simulink model "waterTankBurner"  (R2014b)
settings: Solver=ode1  StartTime=0.0  StopTime=100  FixedStep=0.0001  MaxStep=0.0001  RelTol=1e-3
(part 3 of 4)

== matlab function waterTankBurner/waterTank4/MATLAB Function ==
  data: q input; ON input; OFF input; x input; qNext output; reset output


function [qNext,reset]  = phi(q,  ON, OFF,x)
%#codegen


if q==1 % q=1, tank is in t1
    if ON==0
        qNext=1;
        reset=0;
    elseif ON==1
        qNext=2;
        reset=1;
    else
        qNext=-1;
        reset=-1;
    end;
    
elseif q==2 % q=2, tank is in t2
    if x<100 && OFF==0
        qNext=2;
        reset=0;
    elseif x>=100
        qNext=3;
        reset=1;
    elseif x<100 && OFF==1
        qNext=4;
        reset=1;
    else
        qNext=-1;
        reset=-1;
    end;

elseif q==3 % q=3, tank is in state t3
    if OFF==0
        qNext=3;
        reset=0;
    elseif OFF==1
        qNext=4;
        reset=1;
    else
        qNext=-1;
        reset=-1;
    end;
elseif q==4 % q=4, tank is in state t4
    if x>20 && ON==0
        qNext=4;
        reset=0;
    elseif x<=20
        qNext=1;
        reset=1;
    elseif x>20 && ON==1
        qNext=2;
        reset=1;
    else
        qNext=-1;
        reset=-1;
    end;
else
    qNext=-1; %this should never execute
    reset=-1;%this should never execute
end

== matlab function waterTankBurner/waterTank4/MATLAB Function1 ==
  data: x input; ode1 output; ode2 output; ode3 output; ode4 output
function [ode1,ode2,ode3,ode4] = ODEs(x)
%#codegen
K=0.075;
h=150;
ode1=0;
ode2=K*(h-x);
ode3=0;
ode4=-K*x;

== matlab function waterTankBurner/waterTank5/MATLAB Function ==
  data: q input; ON input; OFF input; x input; qNext output; reset output


function [qNext,reset]  = phi(q,  ON, OFF,x)
%#codegen


if q==1 % q=1, tank is in t1
    if ON==0
        qNext=1;
        reset=0;
    elseif ON==1
        qNext=2;
        reset=1;
    else
        qNext=-1;
        reset=-1;
    end;
    
elseif q==2 % q=2, tank is in t2
    if x<100 && OFF==0
        qNext=2;
        reset=0;
    elseif x>=100
        qNext=3;
        reset=1;
    elseif x<100 && OFF==1
        qNext=4;
        reset=1;
    else
        qNext=-1;
        reset=-1;
    end;

elseif q==3 % q=3, tank is in state t3
    if OFF==0
        qNext=3;
        reset=0;
    elseif OFF==1
        qNext=4;
        reset=1;
    else
        qNext=-1;
        reset=-1;
    end;
elseif q==4 % q=4, tank is in state t4
    if x>20 && ON==0
        qNext=4;
        reset=0;
    elseif x<=20
        qNext=1;
        reset=1;
    elseif x>20 && ON==1
        qNext=2;
        reset=1;
    else
        qNext=-1;
        reset=-1;
    end;
else
    qNext=-1; %this should never execute
    reset=-1;%this should never execute
end

== matlab function waterTankBurner/waterTank5/MATLAB Function1 ==
  data: x input; ode1 output; ode2 output; ode3 output; ode4 output
function [ode1,ode2,ode3,ode4] = ODEs(x)
%#codegen
K=0.075;
h=150;
ode1=0;
ode2=K*(h-x);
ode3=0;
ode4=-K*x;

== matlab function waterTankBurner/waterTank6/MATLAB Function ==
  data: q input; ON input; OFF input; x input; qNext output; reset output


function [qNext,reset]  = phi(q,  ON, OFF,x)
%#codegen


if q==1 % q=1, tank is in t1
    if ON==0
        qNext=1;
        reset=0;
    elseif ON==1
        qNext=2;
        reset=1;
    else
        qNext=-1;
        reset=-1;
    end;
    
elseif q==2 % q=2, tank is in t2
    if x<100 && OFF==0
        qNext=2;
        reset=0;
    elseif x>=100
        qNext=3;
        reset=1;
    elseif x<100 && OFF==1
        qNext=4;
        reset=1;
    else
        qNext=-1;
        reset=-1;
    end;

elseif q==3 % q=3, tank is in state t3
    if OFF==0
        qNext=3;
        reset=0;
    elseif OFF==1
        qNext=4;
        reset=1;
    else
        qNext=-1;
        reset=-1;
    end;
elseif q==4 % q=4, tank is in state t4
    if x>20 && ON==0
        qNext=4;
        reset=0;
    elseif x<=20
        qNext=1;
        reset=1;
    elseif x>20 && ON==1
        qNext=2;
        reset=1;
    else
        qNext=-1;
        reset=-1;
    end;
else
    qNext=-1; %this should never execute
    reset=-1;%this should never execute
end

== matlab function waterTankBurner/waterTank6/MATLAB Function1 ==
  data: x input; ode1 output; ode2 output; ode3 output; ode4 output
function [ode1,ode2,ode3,ode4] = ODEs(x)
%#codegen
K=0.075;
h=150;
ode1=0;
ode2=K*(h-x);
ode3=0;
ode4=-K*x;

== matlab function waterTankBurner/waterTank7/MATLAB Function ==
  data: q input; ON input; OFF input; x input; qNext output; reset output


function [qNext,reset]  = phi(q,  ON, OFF,x)
%#codegen


if q==1 % q=1, tank is in t1
    if ON==0
        qNext=1;
        reset=0;
    elseif ON==1
        qNext=2;
        reset=1;
    else
        qNext=-1;
        reset=-1;
    end;
    
elseif q==2 % q=2, tank is in t2
    if x<100 && OFF==0
        qNext=2;
        reset=0;
    elseif x>=100
        qNext=3;
        reset=1;
    elseif x<100 && OFF==1
        qNext=4;
        reset=1;
    else
        qNext=-1;
        reset=-1;
    end;

elseif q==3 % q=3, tank is in state t3
    if OFF==0
        qNext=3;
        reset=0;
    elseif OFF==1
        qNext=4;
        reset=1;
    else
        qNext=-1;
        reset=-1;
    end;
elseif q==4 % q=4, tank is in state t4
    if x>20 && ON==0
        qNext=4;
        reset=0;
    elseif x<=20
        qNext=1;
        reset=1;
    elseif x>20 && ON==1
        qNext=2;
        reset=1;
    else
        qNext=-1;
        reset=-1;
    end;
else
    qNext=-1; %this should never execute
    reset=-1;%this should never execute
end

== matlab function waterTankBurner/waterTank7/MATLAB Function1 ==
  data: x input; ode1 output; ode2 output; ode3 output; ode4 output
function [ode1,ode2,ode3,ode4] = ODEs(x)
%#codegen
K=0.075;
h=150;
ode1=0;
ode2=K*(h-x);
ode3=0;
ode4=-K*x;

== matlab function waterTankBurner/waterTank10/MATLAB Function ==
  data: q input; ON input; OFF input; x input; qNext output; reset output


function [qNext,reset]  = phi(q,  ON, OFF,x)
%#codegen


if q==1 % q=1, tank is in t1
    if ON==0
        qNext=1;
        reset=0;
    elseif ON==1
        qNext=2;
        reset=1;
    else
        qNext=-1;
        reset=-1;
    end;
    
elseif q==2 % q=2, tank is in t2
    if x<100 && OFF==0
        qNext=2;
        reset=0;
    elseif x>=100
        qNext=3;
        reset=1;
    elseif x<100 && OFF==1
        qNext=4;
        reset=1;
    else
        qNext=-1;
        reset=-1;
    end;

elseif q==3 % q=3, tank is in state t3
    if OFF==0
        qNext=3;
        reset=0;
    elseif OFF==1
        qNext=4;
        reset=1;
    else
        qNext=-1;
        reset=-1;
    end;
elseif q==4 % q=4, tank is in state t4
    if x>20 && ON==0
        qNext=4;
        reset=0;
    elseif x<=20
        qNext=1;
        reset=1;
    elseif x>20 && ON==1
        qNext=2;
        reset=1;
    else
        qNext=-1;
        reset=-1;
    end;
else
    qNext=-1; %this should never execute
    reset=-1;%this should never execute
end

== matlab function waterTankBurner/waterTank10/MATLAB Function1 ==
  data: x input; ode1 output; ode2 output; ode3 output; ode4 output
function [ode1,ode2,ode3,ode4] = ODEs(x)
%#codegen
K=0.075;
h=150;
ode1=0;
ode2=K*(h-x);
ode3=0;
ode4=-K*x;

== matlab function waterTankBurner/waterTank11/MATLAB Function ==
  data: q input; ON input; OFF input; x input; qNext output; reset output


function [qNext,reset]  = phi(q,  ON, OFF,x)
%#codegen


if q==1 % q=1, tank is in t1
    if ON==0
        qNext=1;
        reset=0;
    elseif ON==1
        qNext=2;
        reset=1;
    else
        qNext=-1;
        reset=-1;
    end;
    
elseif q==2 % q=2, tank is in t2
    if x<100 && OFF==0
        qNext=2;
        reset=0;
    elseif x>=100
        qNext=3;
        reset=1;
    elseif x<100 && OFF==1
        qNext=4;
        reset=1;
    else
        qNext=-1;
        reset=-1;
    end;

elseif q==3 % q=3, tank is in state t3
    if OFF==0
        qNext=3;
        reset=0;
    elseif OFF==1
        qNext=4;
        reset=1;
    else
        qNext=-1;
        reset=-1;
    end;
elseif q==4 % q=4, tank is in state t4
    if x>20 && ON==0
        qNext=4;
        reset=0;
    elseif x<=20
        qNext=1;
        reset=1;
    elseif x>20 && ON==1
        qNext=2;
        reset=1;
    else
        qNext=-1;
        reset=-1;
    end;
else
    qNext=-1; %this should never execute
    reset=-1;%this should never execute
end

== matlab function waterTankBurner/waterTank11/MATLAB Function1 ==
  data: x input; ode1 output; ode2 output; ode3 output; ode4 output
function [ode1,ode2,ode3,ode4] = ODEs(x)
%#codegen
K=0.075;
h=150;
ode1=0;
ode2=K*(h-x);
ode3=0;
ode4=-K*x;

== matlab function waterTankBurner/waterTank8/MATLAB Function ==
  data: q input; ON input; OFF input; x input; qNext output; reset output


function [qNext,reset]  = phi(q,  ON, OFF,x)
%#codegen


if q==1 % q=1, tank is in t1
    if ON==0
        qNext=1;
        reset=0;
    elseif ON==1
        qNext=2;
        reset=1;
    else
        qNext=-1;
        reset=-1;
    end;
    
elseif q==2 % q=2, tank is in t2
    if x<100 && OFF==0
        qNext=2;
        reset=0;
    elseif x>=100
        qNext=3;
        reset=1;
    elseif x<100 && OFF==1
        qNext=4;
        reset=1;
    else
        qNext=-1;
        reset=-1;
    end;

elseif q==3 % q=3, tank is in state t3
    if OFF==0
        qNext=3;
        reset=0;
    elseif OFF==1
        qNext=4;
        reset=1;
    else
        qNext=-1;
        reset=-1;
    end;
elseif q==4 % q=4, tank is in state t4
    if x>20 && ON==0
        qNext=4;
        reset=0;
    elseif x<=20
        qNext=1;
        reset=1;
    elseif x>20 && ON==1
        qNext=2;
        reset=1;
    else
        qNext=-1;
        reset=-1;
    end;
else
    qNext=-1; %this should never execute
    reset=-1;%this should never execute
end

== matlab function waterTankBurner/waterTank8/MATLAB Function1 ==
  data: x input; ode1 output; ode2 output; ode3 output; ode4 output
function [ode1,ode2,ode3,ode4] = ODEs(x)
%#codegen
K=0.075;
h=150;
ode1=0;
ode2=K*(h-x);
ode3=0;
ode4=-K*x;

== matlab function waterTankBurner/waterTank9/MATLAB Function ==
  data: q input; ON input; OFF input; x input; qNext output; reset output


function [qNext,reset]  = phi(q,  ON, OFF,x)
%#codegen


if q==1 % q=1, tank is in t1
    if ON==0
        qNext=1;
        reset=0;
    elseif ON==1
        qNext=2;
        reset=1;
    else
        qNext=-1;
        reset=-1;
    end;
    
elseif q==2 % q=2, tank is in t2
    if x<100 && OFF==0
        qNext=2;
        reset=0;
    elseif x>=100
        qNext=3;
        reset=1;
    elseif x<100 && OFF==1
        qNext=4;
        reset=1;
    else
        qNext=-1;
        reset=-1;
    end;

elseif q==3 % q=3, tank is in state t3
    if OFF==0
        qNext=3;
        reset=0;
    elseif OFF==1
        qNext=4;
        reset=1;
    else
        qNext=-1;
        reset=-1;
    end;
elseif q==4 % q=4, tank is in state t4
    if x>20 && ON==0
        qNext=4;
        reset=0;
    elseif x<=20
        qNext=1;
        reset=1;
    elseif x>20 && ON==1
        qNext=2;
        reset=1;
    else
        qNext=-1;
        reset=-1;
    end;
else
    qNext=-1; %this should never execute
    reset=-1;%this should never execute
end

== matlab function waterTankBurner/waterTank9/MATLAB Function1 ==
  data: x input; ode1 output; ode2 output; ode3 output; ode4 output
function [ode1,ode2,ode3,ode4] = ODEs(x)
%#codegen
K=0.075;
h=150;
ode1=0;
ode2=K*(h-x);
ode3=0;
ode4=-K*x;

== matlab function waterTankBurner/waterTank12/MATLAB Function ==
  data: q input; ON input; OFF input; x input; qNext output; reset output


function [qNext,reset]  = phi(q,  ON, OFF,x)
%#codegen


if q==1 % q=1, tank is in t1
    if ON==0
        qNext=1;
        reset=0;
    elseif ON==1
        qNext=2;
        reset=1;
    else
        qNext=-1;
        reset=-1;
    end;
    
elseif q==2 % q=2, tank is in t2
    if x<100 && OFF==0
        qNext=2;
        reset=0;
    elseif x>=100
        qNext=3;
        reset=1;
    elseif x<100 && OFF==1
        qNext=4;
        reset=1;
    else
        qNext=-1;
        reset=-1;
    end;

elseif q==3 % q=3, tank is in state t3
    if OFF==0
        qNext=3;
        reset=0;
    elseif OFF==1
        qNext=4;
        reset=1;
    else
        qNext=-1;
        reset=-1;
    end;
elseif q==4 % q=4, tank is in state t4
    if x>20 && ON==0
        qNext=4;
        reset=0;
    elseif x<=20
        qNext=1;
        reset=1;
    elseif x>20 && ON==1
        qNext=2;
        reset=1;
    else
        qNext=-1;
        reset=-1;
    end;
else
    qNext=-1; %this should never execute
    reset=-1;%this should never execute
end

== matlab function waterTankBurner/waterTank12/MATLAB Function1 ==
  data: x input; ode1 output; ode2 output; ode3 output; ode4 output
function [ode1,ode2,ode3,ode4] = ODEs(x)
%#codegen
K=0.075;
h=150;
ode1=0;
ode2=K*(h-x);
ode3=0;
ode4=-K*x;

== matlab function waterTankBurner/waterTank13/MATLAB Function ==
  data: q input; ON input; OFF input; x input; qNext output; reset output


function [qNext,reset]  = phi(q,  ON, OFF,x)
%#codegen


if q==1 % q=1, tank is in t1
    if ON==0
        qNext=1;
        reset=0;
    elseif ON==1
        qNext=2;
        reset=1;
    else
        qNext=-1;
        reset=-1;
    end;
    
elseif q==2 % q=2, tank is in t2
    if x<100 && OFF==0
        qNext=2;
        reset=0;
    elseif x>=100
        qNext=3;
        reset=1;
    elseif x<100 && OFF==1
        qNext=4;
        reset=1;
    else
        qNext=-1;
        reset=-1;
    end;

elseif q==3 % q=3, tank is in state t3
    if OFF==0
        qNext=3;
        reset=0;
    elseif OFF==1
        qNext=4;
        reset=1;
    else
        qNext=-1;
        reset=-1;
    end;
elseif q==4 % q=4, tank is in state t4
    if x>20 && ON==0
        qNext=4;
        reset=0;
    elseif x<=20
        qNext=1;
        reset=1;
    elseif x>20 && ON==1
        qNext=2;
        reset=1;
    else
        qNext=-1;
        reset=-1;
    end;
else
    qNext=-1; %this should never execute
    reset=-1;%this should never execute
end

== matlab function waterTankBurner/waterTank13/MATLAB Function1 ==
  data: x input; ode1 output; ode2 output; ode3 output; ode4 output
function [ode1,ode2,ode3,ode4] = ODEs(x)
%#codegen
K=0.075;
h=150;
ode1=0;
ode2=K*(h-x);
ode3=0;
ode4=-K*x;

== matlab function waterTankBurner/waterTank14/MATLAB Function ==
  data: q input; ON input; OFF input; x input; qNext output; reset output


function [qNext,reset]  = phi(q,  ON, OFF,x)
%#codegen


if q==1 % q=1, tank is in t1
    if ON==0
        qNext=1;
        reset=0;
    elseif ON==1
        qNext=2;
        reset=1;
    else
        qNext=-1;
        reset=-1;
    end;
    
elseif q==2 % q=2, tank is in t2
    if x<100 && OFF==0
        qNext=2;
        reset=0;
    elseif x>=100
        qNext=3;
        reset=1;
    elseif x<100 && OFF==1
        qNext=4;
        reset=1;
    else
        qNext=-1;
        reset=-1;
    end;

elseif q==3 % q=3, tank is in state t3
    if OFF==0
        qNext=3;
        reset=0;
    elseif OFF==1
        qNext=4;
        reset=1;
    else
        qNext=-1;
        reset=-1;
    end;
elseif q==4 % q=4, tank is in state t4
    if x>20 && ON==0
        qNext=4;
        reset=0;
    elseif x<=20
        qNext=1;
        reset=1;
    elseif x>20 && ON==1
        qNext=2;
        reset=1;
    else
        qNext=-1;
        reset=-1;
    end;
else
    qNext=-1; %this should never execute
    reset=-1;%this should never execute
end

== matlab function waterTankBurner/waterTank14/MATLAB Function1 ==
  data: x input; ode1 output; ode2 output; ode3 output; ode4 output
function [ode1,ode2,ode3,ode4] = ODEs(x)
%#codegen
K=0.075;
h=150;
ode1=0;
ode2=K*(h-x);
ode3=0;
ode4=-K*x;

== matlab function waterTankBurner/waterTank15/MATLAB Function ==
  data: q input; ON input; OFF input; x input; qNext output; reset output


function [qNext,reset]  = phi(q,  ON, OFF,x)
%#codegen


if q==1 % q=1, tank is in t1
    if ON==0
        qNext=1;
        reset=0;
    elseif ON==1
        qNext=2;
        reset=1;
    else
        qNext=-1;
        reset=-1;
    end;
    
elseif q==2 % q=2, tank is in t2
    if x<100 && OFF==0
        qNext=2;
        reset=0;
    elseif x>=100
        qNext=3;
        reset=1;
    elseif x<100 && OFF==1
        qNext=4;
        reset=1;
    else
        qNext=-1;
        reset=-1;
    end;

elseif q==3 % q=3, tank is in state t3
    if OFF==0
        qNext=3;
        reset=0;
    elseif OFF==1
        qNext=4;
        reset=1;
    else
        qNext=-1;
        reset=-1;
    end;
elseif q==4 % q=4, tank is in state t4
    if x>20 && ON==0
        qNext=4;
        reset=0;
    elseif x<=20
        qNext=1;
        reset=1;
    elseif x>20 && ON==1
        qNext=2;
        reset=1;
    else
        qNext=-1;
        reset=-1;
    end;
else
    qNext=-1; %this should never execute
    reset=-1;%this should never execute
end

== matlab function waterTankBurner/waterTank15/MATLAB Function1 ==
  data: x input; ode1 output; ode2 output; ode3 output; ode4 output
function [ode1,ode2,ode3,ode4] = ODEs(x)
%#codegen
K=0.075;
h=150;
ode1=0;
ode2=K*(h-x);
ode3=0;
ode4=-K*x;

== matlab function waterTankBurner/waterTank16/MATLAB Function ==
  data: q input; ON input; OFF input; x input; qNext output; reset output


function [qNext,reset]  = phi(q,  ON, OFF,x)
%#codegen


if q==1 % q=1, tank is in t1
    if ON==0
        qNext=1;
        reset=0;
    elseif ON==1
        qNext=2;
        reset=1;
    else
        qNext=-1;
        reset=-1;
    end;
    
elseif q==2 % q=2, tank is in t2
    if x<100 && OFF==0
        qNext=2;
        reset=0;
    elseif x>=100
        qNext=3;
        reset=1;
    elseif x<100 && OFF==1
        qNext=4;
        reset=1;
    else
        qNext=-1;
        reset=-1;
    end;

elseif q==3 % q=3, tank is in state t3
    if OFF==0
        qNext=3;
        reset=0;
    elseif OFF==1
        qNext=4;
        reset=1;
    else
        qNext=-1;
        reset=-1;
    end;
elseif q==4 % q=4, tank is in state t4
    if x>20 && ON==0
        qNext=4;
        reset=0;
    elseif x<=20
        qNext=1;
        reset=1;
    elseif x>20 && ON==1
        qNext=2;
        reset=1;
    else
        qNext=-1;
        reset=-1;
    end;
else
    qNext=-1; %this should never execute
    reset=-1;%this should never execute
end

== matlab function waterTankBurner/waterTank16/MATLAB Function1 ==
  data: x input; ode1 output; ode2 output; ode3 output; ode4 output
function [ode1,ode2,ode3,ode4] = ODEs(x)
%#codegen
K=0.075;
h=150;
ode1=0;
ode2=K*(h-x);
ode3=0;
ode4=-K*x;

== matlab function waterTankBurner/waterTank17/MATLAB Function ==
  data: q input; ON input; OFF input; x input; qNext output; reset output


function [qNext,reset]  = phi(q,  ON, OFF,x)
%#codegen


if q==1 % q=1, tank is in t1
    if ON==0
        qNext=1;
        reset=0;
    elseif ON==1
        qNext=2;
        reset=1;
    else
        qNext=-1;
        reset=-1;
    end;
    
elseif q==2 % q=2, tank is in t2
    if x<100 && OFF==0
        qNext=2;
        reset=0;
    elseif x>=100
        qNext=3;
        reset=1;
    elseif x<100 && OFF==1
        qNext=4;
        reset=1;
    else
        qNext=-1;
        reset=-1;
    end;

elseif q==3 % q=3, tank is in state t3
    if OFF==0
        qNext=3;
        reset=0;
    elseif OFF==1
        qNext=4;
        reset=1;
    else
        qNext=-1;
        reset=-1;
    end;
elseif q==4 % q=4, tank is in state t4
    if x>20 && ON==0
        qNext=4;
        reset=0;
    elseif x<=20
        qNext=1;
        reset=1;
    elseif x>20 && ON==1
        qNext=2;
        reset=1;
    else
        qNext=-1;
        reset=-1;
    end;
else
    qNext=-1; %this should never execute
    reset=-1;%this should never execute
end

== matlab function waterTankBurner/waterTank17/MATLAB Function1 ==
  data: x input; ode1 output; ode2 output; ode3 output; ode4 output
function [ode1,ode2,ode3,ode4] = ODEs(x)
%#codegen
K=0.075;
h=150;
ode1=0;
ode2=K*(h-x);
ode3=0;
ode4=-K*x;

== matlab function waterTankBurner/waterTank18/MATLAB Function ==
  data: q input; ON input; OFF input; x input; qNext output; reset output


function [qNext,reset]  = phi(q,  ON, OFF,x)
%#codegen


if q==1 % q=1, tank is in t1
    if ON==0
        qNext=1;
        reset=0;
    elseif ON==1
        qNext=2;
        reset=1;
    else
        qNext=-1;
        reset=-1;
    end;
    
elseif q==2 % q=2, tank is in t2
    if x<100 && OFF==0
        qNext=2;
        reset=0;
    elseif x>=100
        qNext=3;
        reset=1;
    elseif x<100 && OFF==1
        qNext=4;
        reset=1;
    else
        qNext=-1;
        reset=-1;
    end;

elseif q==3 % q=3, tank is in state t3
    if OFF==0
        qNext=3;
        reset=0;
    elseif OFF==1
        qNext=4;
        reset=1;
    else
        qNext=-1;
        reset=-1;
    end;
elseif q==4 % q=4, tank is in state t4
    if x>20 && ON==0
        qNext=4;
        reset=0;
    elseif x<=20
        qNext=1;
        reset=1;
    elseif x>20 && ON==1
        qNext=2;
        reset=1;
    else
        qNext=-1;
        reset=-1;
    end;
else
    qNext=-1; %this should never execute
    reset=-1;%this should never execute
end

== matlab function waterTankBurner/waterTank18/MATLAB Function1 ==
  data: x input; ode1 output; ode2 output; ode3 output; ode4 output
function [ode1,ode2,ode3,ode4] = ODEs(x)
%#codegen
K=0.075;
h=150;
ode1=0;
ode2=K*(h-x);
ode3=0;
ode4=-K*x;

== matlab function waterTankBurner/waterTank19/MATLAB Function ==
  data: q input; ON input; OFF input; x input; qNext output; reset output


function [qNext,reset]  = phi(q,  ON, OFF,x)
%#codegen


if q==1 % q=1, tank is in t1
    if ON==0
        qNext=1;
        reset=0;
    elseif ON==1
        qNext=2;
        reset=1;
    else
        qNext=-1;
        reset=-1;
    end;
    
elseif q==2 % q=2, tank is in t2
    if x<100 && OFF==0
        qNext=2;
        reset=0;
    elseif x>=100
        qNext=3;
        reset=1;
    elseif x<100 && OFF==1
        qNext=4;
        reset=1;
    else
        qNext=-1;
        reset=-1;
    end;

elseif q==3 % q=3, tank is in state t3
    if OFF==0
        qNext=3;
        reset=0;
    elseif OFF==1
        qNext=4;
        reset=1;
    else
        qNext=-1;
        reset=-1;
    end;
elseif q==4 % q=4, tank is in state t4
    if x>20 && ON==0
        qNext=4;
        reset=0;
    elseif x<=20
        qNext=1;
        reset=1;
    elseif x>20 && ON==1
        qNext=2;
        reset=1;
    else
        qNext=-1;
        reset=-1;
    end;
else
    qNext=-1; %this should never execute
    reset=-1;%this should never execute
end

== matlab function waterTankBurner/waterTank19/MATLAB Function1 ==
  data: x input; ode1 output; ode2 output; ode3 output; ode4 output
function [ode1,ode2,ode3,ode4] = ODEs(x)
%#codegen
K=0.075;
h=150;
ode1=0;
ode2=K*(h-x);
ode3=0;
ode4=-K*x;

== matlab function waterTankBurner/waterTank20/MATLAB Function ==
  data: q input; ON input; OFF input; x input; qNext output; reset output


function [qNext,reset]  = phi(q,  ON, OFF,x)
%#codegen


if q==1 % q=1, tank is in t1
    if ON==0
        qNext=1;
        reset=0;
    elseif ON==1
        qNext=2;
        reset=1;
    else
        qNext=-1;
        reset=-1;
    end;
    
elseif q==2 % q=2, tank is in t2
    if x<100 && OFF==0
        qNext=2;
        reset=0;
    elseif x>=100
        qNext=3;
        reset=1;
    elseif x<100 && OFF==1
        qNext=4;
        reset=1;
    else
        qNext=-1;
        reset=-1;
    end;

elseif q==3 % q=3, tank is in state t3
    if OFF==0
        qNext=3;
        reset=0;
    elseif OFF==1
        qNext=4;
        reset=1;
    else
        qNext=-1;
        reset=-1;
    end;
elseif q==4 % q=4, tank is in state t4
    if x>20 && ON==0
        qNext=4;
        reset=0;
    elseif x<=20
        qNext=1;
        reset=1;
    elseif x>20 && ON==1
        qNext=2;
        reset=1;
    else
        qNext=-1;
        reset=-1;
    end;
else
    qNext=-1; %this should never execute
    reset=-1;%this should never execute
end

== matlab function waterTankBurner/waterTank20/MATLAB Function1 ==
  data: x input; ode1 output; ode2 output; ode3 output; ode4 output
function [ode1,ode2,ode3,ode4] = ODEs(x)
%#codegen
K=0.075;
h=150;
ode1=0;
ode2=K*(h-x);
ode3=0;
ode4=-K*x;

== matlab function waterTankBurner/waterTank21/MATLAB Function ==
  data: q input; ON input; OFF input; x input; qNext output; reset output


function [qNext,reset]  = phi(q,  ON, OFF,x)
%#codegen


if q==1 % q=1, tank is in t1
    if ON==0
        qNext=1;
        reset=0;
    elseif ON==1
        qNext=2;
        reset=1;
    else
        qNext=-1;
        reset=-1;
    end;
    
elseif q==2 % q=2, tank is in t2
    if x<100 && OFF==0
        qNext=2;
        reset=0;
    elseif x>=100
        qNext=3;
        reset=1;
    elseif x<100 && OFF==1
        qNext=4;
        reset=1;
    else
        qNext=-1;
        reset=-1;
    end;

elseif q==3 % q=3, tank is in state t3
    if OFF==0
        qNext=3;
        reset=0;
    elseif OFF==1
        qNext=4;
        reset=1;
    else
        qNext=-1;
        reset=-1;
    end;
elseif q==4 % q=4, tank is in state t4
    if x>20 && ON==0
        qNext=4;
        reset=0;
    elseif x<=20
        qNext=1;
        reset=1;
    elseif x>20 && ON==1
        qNext=2;
        reset=1;
    else
        qNext=-1;
        reset=-1;
    end;
else
    qNext=-1; %this should never execute
    reset=-1;%this should never execute
end

== matlab function waterTankBurner/waterTank21/MATLAB Function1 ==
  data: x input; ode1 output; ode2 output; ode3 output; ode4 output
function [ode1,ode2,ode3,ode4] = ODEs(x)
%#codegen
K=0.075;
h=150;
ode1=0;
ode2=K*(h-x);
ode3=0;
ode4=-K*x;

== matlab function waterTankBurner/waterTank22/MATLAB Function ==
  data: q input; ON input; OFF input; x input; qNext output; reset output


function [qNext,reset]  = phi(q,  ON, OFF,x)
%#codegen


if q==1 % q=1, tank is in t1
    if ON==0
        qNext=1;
        reset=0;
    elseif ON==1
        qNext=2;
        reset=1;
    else
        qNext=-1;
        reset=-1;
    end;
    
elseif q==2 % q=2, tank is in t2
    if x<100 && OFF==0
        qNext=2;
        reset=0;
    elseif x>=100
        qNext=3;
        reset=1;
    elseif x<100 && OFF==1
        qNext=4;
        reset=1;
    else
        qNext=-1;
        reset=-1;
    end;

elseif q==3 % q=3, tank is in state t3
    if OFF==0
        qNext=3;
        reset=0;
    elseif OFF==1
        qNext=4;
        reset=1;
    else
        qNext=-1;
        reset=-1;
    end;
elseif q==4 % q=4, tank is in state t4
    if x>20 && ON==0
        qNext=4;
        reset=0;
    elseif x<=20
        qNext=1;
        reset=1;
    elseif x>20 && ON==1
        qNext=2;
        reset=1;
    else
        qNext=-1;
        reset=-1;
    end;
else
    qNext=-1; %this should never execute
    reset=-1;%this should never execute
end

== matlab function waterTankBurner/waterTank22/MATLAB Function1 ==
  data: x input; ode1 output; ode2 output; ode3 output; ode4 output
function [ode1,ode2,ode3,ode4] = ODEs(x)
%#codegen
K=0.075;
h=150;
ode1=0;
ode2=K*(h-x);
ode3=0;
ode4=-K*x;

== matlab function waterTankBurner/waterTank23/MATLAB Function ==
  data: q input; ON input; OFF input; x input; qNext output; reset output


function [qNext,reset]  = phi(q,  ON, OFF,x)
%#codegen


if q==1 % q=1, tank is in t1
    if ON==0
        qNext=1;
        reset=0;
    elseif ON==1
        qNext=2;
        reset=1;
    else
        qNext=-1;
        reset=-1;
    end;
    
elseif q==2 % q=2, tank is in t2
    if x<100 && OFF==0
        qNext=2;
        reset=0;
    elseif x>=100
        qNext=3;
        reset=1;
    elseif x<100 && OFF==1
        qNext=4;
        reset=1;
    else
        qNext=-1;
        reset=-1;
    end;

elseif q==3 % q=3, tank is in state t3
    if OFF==0
        qNext=3;
        reset=0;
    elseif OFF==1
        qNext=4;
        reset=1;
    else
        qNext=-1;
        reset=-1;
    end;
elseif q==4 % q=4, tank is in state t4
    if x>20 && ON==0
        qNext=4;
        reset=0;
    elseif x<=20
        qNext=1;
        reset=1;
    elseif x>20 && ON==1
        qNext=2;
        reset=1;
    else
        qNext=-1;
        reset=-1;
    end;
else
    qNext=-1; %this should never execute
    reset=-1;%this should never execute
end

== matlab function waterTankBurner/waterTank23/MATLAB Function1 ==
  data: x input; ode1 output; ode2 output; ode3 output; ode4 output
function [ode1,ode2,ode3,ode4] = ODEs(x)
%#codegen
K=0.075;
h=150;
ode1=0;
ode2=K*(h-x);
ode3=0;
ode4=-K*x;

== matlab function waterTankBurner/waterTank24/MATLAB Function ==
  data: q input; ON input; OFF input; x input; qNext output; reset output


function [qNext,reset]  = phi(q,  ON, OFF,x)
%#codegen


if q==1 % q=1, tank is in t1
    if ON==0
        qNext=1;
        reset=0;
    elseif ON==1
        qNext=2;
        reset=1;
    else
        qNext=-1;
        reset=-1;
    end;
    
elseif q==2 % q=2, tank is in t2
    if x<100 && OFF==0
        qNext=2;
        reset=0;
    elseif x>=100
        qNext=3;
        reset=1;
    elseif x<100 && OFF==1
        qNext=4;
        reset=1;
    else
        qNext=-1;
        reset=-1;
    end;

elseif q==3 % q=3, tank is in state t3
    if OFF==0
        qNext=3;
        reset=0;
    elseif OFF==1
        qNext=4;
        reset=1;
    else
        qNext=-1;
        reset=-1;
    end;
elseif q==4 % q=4, tank is in state t4
    if x>20 && ON==0
        qNext=4;
        reset=0;
    elseif x<=20
        qNext=1;
        reset=1;
    elseif x>20 && ON==1
        qNext=2;
        reset=1;
    else
        qNext=-1;
        reset=-1;
    end;
else
    qNext=-1; %this should never execute
    reset=-1;%this should never execute
end

== matlab function waterTankBurner/waterTank24/MATLAB Function1 ==
  data: x input; ode1 output; ode2 output; ode3 output; ode4 output
function [ode1,ode2,ode3,ode4] = ODEs(x)
%#codegen
K=0.075;
h=150;
ode1=0;
ode2=K*(h-x);
ode3=0;
ode4=-K*x;

== matlab function waterTankBurner/waterTank25/MATLAB Function ==
  data: q input; ON input; OFF input; x input; qNext output; reset output


function [qNext,reset]  = phi(q,  ON, OFF,x)
%#codegen


if q==1 % q=1, tank is in t1
    if ON==0
        qNext=1;
        reset=0;
    elseif ON==1
        qNext=2;
        reset=1;
    else
        qNext=-1;
        reset=-1;
    end;
    
elseif q==2 % q=2, tank is in t2
    if x<100 && OFF==0
        qNext=2;
        reset=0;
    elseif x>=100
        qNext=3;
        reset=1;
    elseif x<100 && OFF==1
        qNext=4;
        reset=1;
    else
        qNext=-1;
        reset=-1;
    end;

elseif q==3 % q=3, tank is in state t3
    if OFF==0
        qNext=3;
        reset=0;
    elseif OFF==1
        qNext=4;
        reset=1;
    else
        qNext=-1;
        reset=-1;
    end;
elseif q==4 % q=4, tank is in state t4
    if x>20 && ON==0
        qNext=4;
        reset=0;
    elseif x<=20
        qNext=1;
        reset=1;
    elseif x>20 && ON==1
        qNext=2;
        reset=1;
    else
        qNext=-1;
        reset=-1;
    end;
else
    qNext=-1; %this should never execute
    reset=-1;%this should never execute
end

== matlab function waterTankBurner/waterTank25/MATLAB Function1 ==
  data: x input; ode1 output; ode2 output; ode3 output; ode4 output
function [ode1,ode2,ode3,ode4] = ODEs(x)
%#codegen
K=0.075;
h=150;
ode1=0;
ode2=K*(h-x);
ode3=0;
ode4=-K*x;

== matlab function waterTankBurner/waterTank26/MATLAB Function ==
  data: q input; ON input; OFF input; x input; qNext output; reset output


function [qNext,reset]  = phi(q,  ON, OFF,x)
%#codegen


if q==1 % q=1, tank is in t1
    if ON==0
        qNext=1;
        reset=0;
    elseif ON==1
        qNext=2;
        reset=1;
    else
        qNext=-1;
        reset=-1;
    end;
    
elseif q==2 % q=2, tank is in t2
    if x<100 && OFF==0
        qNext=2;
        reset=0;
    elseif x>=100
        qNext=3;
        reset=1;
    elseif x<100 && OFF==1
        qNext=4;
        reset=1;
    else
        qNext=-1;
        reset=-1;
    end;

elseif q==3 % q=3, tank is in state t3
    if OFF==0
        qNext=3;
        reset=0;
    elseif OFF==1
        qNext=4;
        reset=1;
    else
        qNext=-1;
        reset=-1;
    end;
elseif q==4 % q=4, tank is in state t4
    if x>20 && ON==0
        qNext=4;
        reset=0;
    elseif x<=20
        qNext=1;
        reset=1;
    elseif x>20 && ON==1
        qNext=2;
        reset=1;
    else
        qNext=-1;
        reset=-1;
    end;
else
    qNext=-1; %this should never execute
    reset=-1;%this should never execute
end

== matlab function waterTankBurner/waterTank26/MATLAB Function1 ==
  data: x input; ode1 output; ode2 output; ode3 output; ode4 output
function [ode1,ode2,ode3,ode4] = ODEs(x)
%#codegen
K=0.075;
h=150;
ode1=0;
ode2=K*(h-x);
ode3=0;
ode4=-K*x;

== matlab function waterTankBurner/waterTank27/MATLAB Function ==
  data: q input; ON input; OFF input; x input; qNext output; reset output


function [qNext,reset]  = phi(q,  ON, OFF,x)
%#codegen


if q==1 % q=1, tank is in t1
    if ON==0
        qNext=1;
        reset=0;
    elseif ON==1
        qNext=2;
        reset=1;
    else
        qNext=-1;
        reset=-1;
    end;
    
elseif q==2 % q=2, tank is in t2
    if x<100 && OFF==0
        qNext=2;
        reset=0;
    elseif x>=100
        qNext=3;
        reset=1;
    elseif x<100 && OFF==1
        qNext=4;
        reset=1;
    else
        qNext=-1;
        reset=-1;
    end;

elseif q==3 % q=3, tank is in state t3
    if OFF==0
        qNext=3;
        reset=0;
    elseif OFF==1
        qNext=4;
        reset=1;
    else
        qNext=-1;
        reset=-1;
    end;
elseif q==4 % q=4, tank is in state t4
    if x>20 && ON==0
        qNext=4;
        reset=0;
    elseif x<=20
        qNext=1;
        reset=1;
    elseif x>20 && ON==1
        qNext=2;
        reset=1;
    else
        qNext=-1;
        reset=-1;
    end;
else
    qNext=-1; %this should never execute
    reset=-1;%this should never execute
end

== matlab function waterTankBurner/waterTank27/MATLAB Function1 ==
  data: x input; ode1 output; ode2 output; ode3 output; ode4 output
function [ode1,ode2,ode3,ode4] = ODEs(x)
%#codegen
K=0.075;
h=150;
ode1=0;
ode2=K*(h-x);
ode3=0;
ode4=-K*x;

== matlab function waterTankBurner/waterTank28/MATLAB Function ==
  data: q input; ON input; OFF input; x input; qNext output; reset output


function [qNext,reset]  = phi(q,  ON, OFF,x)
%#codegen


if q==1 % q=1, tank is in t1
    if ON==0
        qNext=1;
        reset=0;
    elseif ON==1
        qNext=2;
        reset=1;
    else
        qNext=-1;
        reset=-1;
    end;
    
elseif q==2 % q=2, tank is in t2
    if x<100 && OFF==0
        qNext=2;
        reset=0;
    elseif x>=100
        qNext=3;
        reset=1;
    elseif x<100 && OFF==1
        qNext=4;
        reset=1;
    else
        qNext=-1;
        reset=-1;
    end;

elseif q==3 % q=3, tank is in state t3
    if OFF==0
        qNext=3;
        reset=0;
    elseif OFF==1
        qNext=4;
        reset=1;
    else
        qNext=-1;
        reset=-1;
    end;
elseif q==4 % q=4, tank is in state t4
    if x>20 && ON==0
        qNext=4;
        reset=0;
    elseif x<=20
        qNext=1;
        reset=1;
    elseif x>20 && ON==1
        qNext=2;
        reset=1;
    else
        qNext=-1;
        reset=-1;
    end;
else
    qNext=-1; %this should never execute
    reset=-1;%this should never execute
end

== matlab function waterTankBurner/waterTank28/MATLAB Function1 ==
  data: x input; ode1 output; ode2 output; ode3 output; ode4 output
function [ode1,ode2,ode3,ode4] = ODEs(x)
%#codegen
K=0.075;
h=150;
ode1=0;
ode2=K*(h-x);
ode3=0;
ode4=-K*x;

== matlab function waterTankBurner/waterTank29/MATLAB Function ==
  data: q input; ON input; OFF input; x input; qNext output; reset output


function [qNext,reset]  = phi(q,  ON, OFF,x)
%#codegen


if q==1 % q=1, tank is in t1
    if ON==0
        qNext=1;
        reset=0;
    elseif ON==1
        qNext=2;
        reset=1;
    else
        qNext=-1;
        reset=-1;
    end;
    
elseif q==2 % q=2, tank is in t2
    if x<100 && OFF==0
        qNext=2;
        reset=0;
    elseif x>=100
        qNext=3;
        reset=1;
    elseif x<100 && OFF==1
        qNext=4;
        reset=1;
    else
        qNext=-1;
        reset=-1;
    end;

elseif q==3 % q=3, tank is in state t3
    if OFF==0
        qNext=3;
        reset=0;
    elseif OFF==1
        qNext=4;
        reset=1;
    else
        qNext=-1;
        reset=-1;
    end;
elseif q==4 % q=4, tank is in state t4
    if x>20 && ON==0
        qNext=4;
        reset=0;
    elseif x<=20
        qNext=1;
        reset=1;
    elseif x>20 && ON==1
        qNext=2;
        reset=1;
    else
        qNext=-1;
        reset=-1;
    end;
else
    qNext=-1; %this should never execute
    reset=-1;%this should never execute
end

== matlab function waterTankBurner/waterTank29/MATLAB Function1 ==
  data: x input; ode1 output; ode2 output; ode3 output; ode4 output
function [ode1,ode2,ode3,ode4] = ODEs(x)
%#codegen
K=0.075;
h=150;
ode1=0;
ode2=K*(h-x);
ode3=0;
ode4=-K*x;

== matlab function waterTankBurner/waterTank30/MATLAB Function ==
  data: q input; ON input; OFF input; x input; qNext output; reset output


function [qNext,reset]  = phi(q,  ON, OFF,x)
%#codegen


if q==1 % q=1, tank is in t1
    if ON==0
        qNext=1;
        reset=0;
    elseif ON==1
        qNext=2;
        reset=1;
    else
        qNext=-1;
        reset=-1;
    end;
    
elseif q==2 % q=2, tank is in t2
    if x<100 && OFF==0
        qNext=2;
        reset=0;
    elseif x>=100
        qNext=3;
        reset=1;
    elseif x<100 && OFF==1
        qNext=4;
        reset=1;
    else
        qNext=-1;
        reset=-1;
    end;

elseif q==3 % q=3, tank is in state t3
    if OFF==0
        qNext=3;
        reset=0;
    elseif OFF==1
        qNext=4;
        reset=1;
    else
        qNext=-1;
        reset=-1;
    end;
elseif q==4 % q=4, tank is in state t4
    if x>20 && ON==0
        qNext=4;
        reset=0;
    elseif x<=20
        qNext=1;
        reset=1;
    elseif x>20 && ON==1
        qNext=2;
        reset=1;
    else
        qNext=-1;
        reset=-1;
    end;
else
    qNext=-1; %this should never execute
    reset=-1;%this should never execute
end

== matlab function waterTankBurner/waterTank30/MATLAB Function1 ==
  data: x input; ode1 output; ode2 output; ode3 output; ode4 output
function [ode1,ode2,ode3,ode4] = ODEs(x)
%#codegen
K=0.075;
h=150;
ode1=0;
ode2=K*(h-x);
ode3=0;
ode4=-K*x;

== matlab function waterTankBurner/waterTank31/MATLAB Function ==
  data: q input; ON input; OFF input; x input; qNext output; reset output


function [qNext,reset]  = phi(q,  ON, OFF,x)
%#codegen


if q==1 % q=1, tank is in t1
    if ON==0
        qNext=1;
        reset=0;
    elseif ON==1
        qNext=2;
        reset=1;
    else
        qNext=-1;
        reset=-1;
    end;
    
elseif q==2 % q=2, tank is in t2
    if x<100 && OFF==0
        qNext=2;
        reset=0;
    elseif x>=100
        qNext=3;
        reset=1;
    elseif x<100 && OFF==1
        qNext=4;
        reset=1;
    else
        qNext=-1;
        reset=-1;
    end;

elseif q==3 % q=3, tank is in state t3
    if OFF==0
        qNext=3;
        reset=0;
    elseif OFF==1
        qNext=4;
        reset=1;
    else
        qNext=-1;
        reset=-1;
    end;
elseif q==4 % q=4, tank is in state t4
    if x>20 && ON==0
        qNext=4;
        reset=0;
    elseif x<=20
        qNext=1;
        reset=1;
    elseif x>20 && ON==1
        qNext=2;
        reset=1;
    else
        qNext=-1;
        reset=-1;
    end;
else
    qNext=-1; %this should never execute
    reset=-1;%this should never execute
end

== matlab function waterTankBurner/waterTank31/MATLAB Function1 ==
  data: x input; ode1 output; ode2 output; ode3 output; ode4 output
function [ode1,ode2,ode3,ode4] = ODEs(x)
%#codegen
K=0.075;
h=150;
ode1=0;
ode2=K*(h-x);
ode3=0;
ode4=-K*x;

== matlab function waterTankBurner/waterTank32/MATLAB Function ==
  data: q input; ON input; OFF input; x input; qNext output; reset output


function [qNext,reset]  = phi(q,  ON, OFF,x)
%#codegen


if q==1 % q=1, tank is in t1
    if ON==0
        qNext=1;
        reset=0;
    elseif ON==1
        qNext=2;
        reset=1;
    else
        qNext=-1;
        reset=-1;
    end;
    
elseif q==2 % q=2, tank is in t2
    if x<100 && OFF==0
        qNext=2;
        reset=0;
    elseif x>=100
        qNext=3;
        reset=1;
    elseif x<100 && OFF==1
        qNext=4;
        reset=1;
    else
        qNext=-1;
        reset=-1;
    end;

elseif q==3 % q=3, tank is in state t3
    if OFF==0
        qNext=3;
        reset=0;
    elseif OFF==1
        qNext=4;
        reset=1;
    else
        qNext=-1;
        reset=-1;
    end;
elseif q==4 % q=4, tank is in state t4
    if x>20 && ON==0
        qNext=4;
        reset=0;
    elseif x<=20
        qNext=1;
        reset=1;
    elseif x>20 && ON==1
        qNext=2;
        reset=1;
    else
        qNext=-1;
        reset=-1;
    end;
else
    qNext=-1; %this should never execute
    reset=-1;%this should never execute
end

== matlab function waterTankBurner/waterTank32/MATLAB Function1 ==
  data: x input; ode1 output; ode2 output; ode3 output; ode4 output
function [ode1,ode2,ode3,ode4] = ODEs(x)
%#codegen
K=0.075;
h=150;
ode1=0;
ode2=K*(h-x);
ode3=0;
ode4=-K*x;

== matlab function waterTankBurner/waterTank33/MATLAB Function ==
  data: q input; ON input; OFF input; x input; qNext output; reset output


function [qNext,reset]  = phi(q,  ON, OFF,x)
%#codegen


if q==1 % q=1, tank is in t1
    if ON==0
        qNext=1;
        reset=0;
    elseif ON==1
        qNext=2;
        reset=1;
    else
        qNext=-1;
        reset=-1;
    end;
    
elseif q==2 % q=2, tank is in t2
    if x<100 && OFF==0
        qNext=2;
        reset=0;
    elseif x>=100
        qNext=3;
        reset=1;
    elseif x<100 && OFF==1
        qNext=4;
        reset=1;
    else
        qNext=-1;
        reset=-1;
    end;

elseif q==3 % q=3, tank is in state t3
    if OFF==0
        qNext=3;
        reset=0;
    elseif OFF==1
        qNext=4;
        reset=1;
    else
        qNext=-1;
        reset=-1;
    end;
elseif q==4 % q=4, tank is in state t4
    if x>20 && ON==0
        qNext=4;
        reset=0;
    elseif x<=20
        qNext=1;
        reset=1;
    elseif x>20 && ON==1
        qNext=2;
        reset=1;
    else
        qNext=-1;
        reset=-1;
    end;
else
    qNext=-1; %this should never execute
    reset=-1;%this should never execute
end

== matlab function waterTankBurner/waterTank33/MATLAB Function1 ==
  data: x input; ode1 output; ode2 output; ode3 output; ode4 output
function [ode1,ode2,ode3,ode4] = ODEs(x)
%#codegen
K=0.075;
h=150;
ode1=0;
ode2=K*(h-x);
ode3=0;
ode4=-K*x;

== matlab function waterTankBurner/waterTank34/MATLAB Function ==
  data: q input; ON input; OFF input; x input; qNext output; reset output


function [qNext,reset]  = phi(q,  ON, OFF,x)
%#codegen


if q==1 % q=1, tank is in t1
    if ON==0
        qNext=1;
        reset=0;
    elseif ON==1
        qNext=2;
        reset=1;
    else
        qNext=-1;
        reset=-1;
    end;
    
elseif q==2 % q=2, tank is in t2
    if x<100 && OFF==0
        qNext=2;
        reset=0;
    elseif x>=100
        qNext=3;
        reset=1;
    elseif x<100 && OFF==1
        qNext=4;
        reset=1;
    else
        qNext=-1;
        reset=-1;
    end;

elseif q==3 % q=3, tank is in state t3
    if OFF==0
        qNext=3;
        reset=0;
    elseif OFF==1
        qNext=4;
        reset=1;
    else
        qNext=-1;
        reset=-1;
    end;
elseif q==4 % q=4, tank is in state t4
    if x>20 && ON==0
        qNext=4;
        reset=0;
    elseif x<=20
        qNext=1;
        reset=1;
    elseif x>20 && ON==1
        qNext=2;
        reset=1;
    else
        qNext=-1;
        reset=-1;
    end;
else
    qNext=-1; %this should never execute
    reset=-1;%this should never execute
end

== matlab function waterTankBurner/waterTank34/MATLAB Function1 ==
  data: x input; ode1 output; ode2 output; ode3 output; ode4 output
function [ode1,ode2,ode3,ode4] = ODEs(x)
%#codegen
K=0.075;
h=150;
ode1=0;
ode2=K*(h-x);
ode3=0;
ode4=-K*x;

== matlab function waterTankBurner/waterTank35/MATLAB Function ==
  data: q input; ON input; OFF input; x input; qNext output; reset output


function [qNext,reset]  = phi(q,  ON, OFF,x)
%#codegen


if q==1 % q=1, tank is in t1
    if ON==0
        qNext=1;
        reset=0;
    elseif ON==1
        qNext=2;
        reset=1;
    else
        qNext=-1;
        reset=-1;
    end;
    
elseif q==2 % q=2, tank is in t2
    if x<100 && OFF==0
        qNext=2;
        reset=0;
    elseif x>=100
        qNext=3;
        reset=1;
    elseif x<100 && OFF==1
        qNext=4;
        reset=1;
    else
        qNext=-1;
        reset=-1;
    end;

elseif q==3 % q=3, tank is in state t3
    if OFF==0
        qNext=3;
        reset=0;
    elseif OFF==1
        qNext=4;
        reset=1;
    else
        qNext=-1;
        reset=-1;
    end;
elseif q==4 % q=4, tank is in state t4
    if x>20 && ON==0
        qNext=4;
        reset=0;
    elseif x<=20
        qNext=1;
        reset=1;
    elseif x>20 && ON==1
        qNext=2;
        reset=1;
    else
        qNext=-1;
        reset=-1;
    end;
else
    qNext=-1; %this should never execute
    reset=-1;%this should never execute
end

== matlab function waterTankBurner/waterTank35/MATLAB Function1 ==
  data: x input; ode1 output; ode2 output; ode3 output; ode4 output
function [ode1,ode2,ode3,ode4] = ODEs(x)
%#codegen
K=0.075;
h=150;
ode1=0;
ode2=K*(h-x);
ode3=0;
ode4=-K*x;

== matlab function waterTankBurner/waterTank36/MATLAB Function ==
  data: q input; ON input; OFF input; x input; qNext output; reset output


function [qNext,reset]  = phi(q,  ON, OFF,x)
%#codegen


if q==1 % q=1, tank is in t1
    if ON==0
        qNext=1;
        reset=0;
    elseif ON==1
        qNext=2;
        reset=1;
    else
        qNext=-1;
        reset=-1;
    end;
    
elseif q==2 % q=2, tank is in t2
    if x<100 && OFF==0
        qNext=2;
        reset=0;
    elseif x>=100
        qNext=3;
        reset=1;
    elseif x<100 && OFF==1
        qNext=4;
        reset=1;
    else
        qNext=-1;
        reset=-1;
    end;

elseif q==3 % q=3, tank is in state t3
    if OFF==0
        qNext=3;
        reset=0;
    elseif OFF==1
        qNext=4;
        reset=1;
    else
        qNext=-1;
        reset=-1;
    end;
elseif q==4 % q=4, tank is in state t4
    if x>20 && ON==0
        qNext=4;
        reset=0;
    elseif x<=20
        qNext=1;
        reset=1;
    elseif x>20 && ON==1
        qNext=2;
        reset=1;
    else
        qNext=-1;
        reset=-1;
    end;
else
    qNext=-1; %this should never execute
    reset=-1;%this should never execute
end

== matlab function waterTankBurner/waterTank36/MATLAB Function1 ==
  data: x input; ode1 output; ode2 output; ode3 output; ode4 output
function [ode1,ode2,ode3,ode4] = ODEs(x)
%#codegen
K=0.075;
h=150;
ode1=0;
ode2=K*(h-x);
ode3=0;
ode4=-K*x;

== matlab function waterTankBurner/waterTank37/MATLAB Function ==
  data: q input; ON input; OFF input; x input; qNext output; reset output


function [qNext,reset]  = phi(q,  ON, OFF,x)
%#codegen


if q==1 % q=1, tank is in t1
    if ON==0
        qNext=1;
        reset=0;
    elseif ON==1
        qNext=2;
        reset=1;
    else
        qNext=-1;
        reset=-1;
    end;
    
elseif q==2 % q=2, tank is in t2
    if x<100 && OFF==0
        qNext=2;
        reset=0;
    elseif x>=100
        qNext=3;
        reset=1;
    elseif x<100 && OFF==1
        qNext=4;
        reset=1;
    else
        qNext=-1;
        reset=-1;
    end;

elseif q==3 % q=3, tank is in state t3
    if OFF==0
        qNext=3;
        reset=0;
    elseif OFF==1
        qNext=4;
        reset=1;
    else
        qNext=-1;
        reset=-1;
    end;
elseif q==4 % q=4, tank is in state t4
    if x>20 && ON==0
        qNext=4;
        reset=0;
    elseif x<=20
        qNext=1;
        reset=1;
    elseif x>20 && ON==1
        qNext=2;
        reset=1;
    else
        qNext=-1;
        reset=-1;
    end;
else
    qNext=-1; %this should never execute
    reset=-1;%this should never execute
end

== matlab function waterTankBurner/waterTank37/MATLAB Function1 ==
  data: x input; ode1 output; ode2 output; ode3 output; ode4 output
function [ode1,ode2,ode3,ode4] = ODEs(x)
%#codegen
K=0.075;
h=150;
ode1=0;
ode2=K*(h-x);
ode3=0;
ode4=-K*x;

== matlab function waterTankBurner/waterTank38/MATLAB Function ==
  data: q input; ON input; OFF input; x input; qNext output; reset output


function [qNext,reset]  = phi(q,  ON, OFF,x)
%#codegen


if q==1 % q=1, tank is in t1
    if ON==0
        qNext=1;
        reset=0;
    elseif ON==1
        qNext=2;
        reset=1;
    else
        qNext=-1;
        reset=-1;
    end;
    
elseif q==2 % q=2, tank is in t2
    if x<100 && OFF==0
        qNext=2;
        reset=0;
    elseif x>=100
        qNext=3;
        reset=1;
    elseif x<100 && OFF==1
        qNext=4;
        reset=1;
    else
        qNext=-1;
        reset=-1;
    end;

elseif q==3 % q=3, tank is in state t3
    if OFF==0
        qNext=3;
        reset=0;
    elseif OFF==1
        qNext=4;
        reset=1;
    else
        qNext=-1;
        reset=-1;
    end;
elseif q==4 % q=4, tank is in state t4
    if x>20 && ON==0
        qNext=4;
        reset=0;
    elseif x<=20
        qNext=1;
        reset=1;
    elseif x>20 && ON==1
        qNext=2;
        reset=1;
    else
        qNext=-1;
        reset=-1;
    end;
else
    qNext=-1; %this should never execute
    reset=-1;%this should never execute
end
